simulink model "q2x2sim"  (R2025b)
settings: Solver=ode45  StartTime=0.0  StopTime=15  MaxStep=.1  RelTol=1e-6  AbsTol=1e-6
model workspace (MAT data in the model file):
  Omega = 0.6
values from neighbouring files (symbols this model uses):
  A = zeros(sum(neqs), 4*NK)    [kernelsc.m]    (also in kernelscinv.m; kernelso.m; kernelsoinv.m; q2x2simu.m = zeros(2*xg))
  Ao = A - [P1; P2]*C    [q2x2simu.m]
  B = zeros(2*xg, 1)    [q2x2simu.m]
  Bo = [[P1; P2] + r*B, B]    [q2x2simu.m]
  C = B'    [q2x2simu.m]
  mu0 = 8    [bounds.m]    (also in histogrametc.m = 10; q2x2simu.m)
  xg = 128    [bounds.m]    (also in q2x2simu.m)
  z0 = [p * v0_ic(x1); v0_ic(x0)]    [histogrametc.m]    (also in q2x2simu.m = [p*v0(x1), v0(x0)]')
  z0hat = 1.5 * z0    [histogrametc.m]    (also in q2x2simu.m = 1.5*z0)
undefined symbols (not defined in the file or in its folder): K1, K2
settings Model: Creator=humaloja  LastModifiedBy=koudohodeflorent

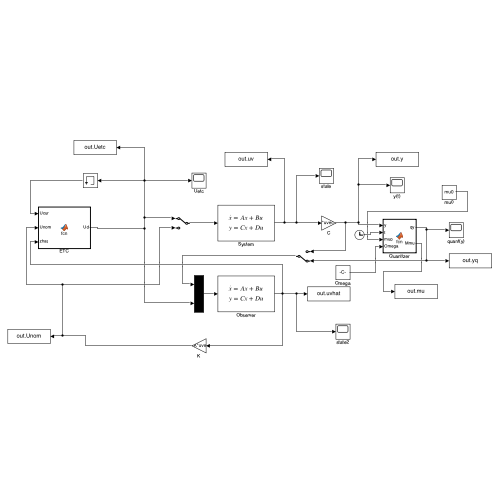
[thumbnail: Simulink's stored preview of the top-level diagram]
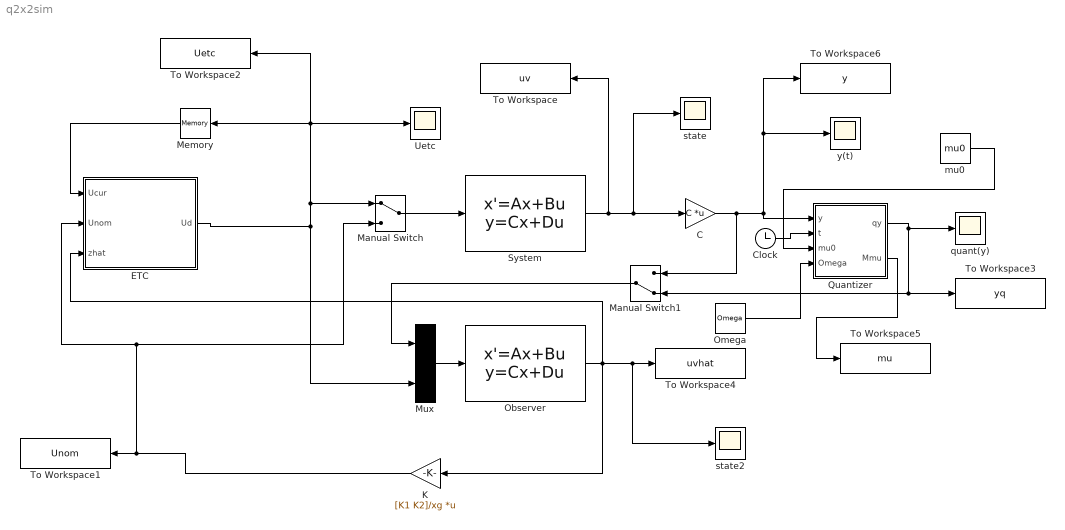
== system q2x2sim ==
  C : Gain  Gain=C  Multiplication=Matrix(K*u) (u vector)
  Clock : Clock
  ETC : MATLAB Function  TreatAsAtomicUnit=on
  K : Gain  Gain=[K1 K2]/xg  Multiplication=Matrix(K*u) (u vector)
  Manual Switch : ManualSwitch
  Manual Switch1 : ManualSwitch  CurrentSetting=0
  Memory : Memory
  Mux : Mux  Inputs=2
  Observer : StateSpace  A=Ao  B=Bo  C=eye(2*xg)  D=zeros(2*xg,2)  InitialCondition=z0hat
  Omega : Constant  Value=Omega
  Quantizer : MATLAB Function  TreatAsAtomicUnit=on
  System : StateSpace  A=A  B=B  C=eye(2*xg)  D=zeros(2*xg,1)  InitialCondition=z0
  To Workspace : ToWorkspace  VariableName=uv  SaveFormat=Timeseries  SampleTime=-1
  To Workspace1 : ToWorkspace  VariableName=Unom  SaveFormat=Timeseries  SampleTime=-1
  To Workspace2 : ToWorkspace  VariableName=Uetc  SaveFormat=Timeseries  SampleTime=-1
  To Workspace3 : ToWorkspace  VariableName=yq  SaveFormat=Timeseries  SampleTime=-1
  To Workspace4 : ToWorkspace  VariableName=uvhat  SaveFormat=Timeseries  SampleTime=-1
  To Workspace5 : ToWorkspace  VariableName=mu  SaveFormat=Timeseries  SampleTime=-1
  To Workspace6 : ToWorkspace  VariableName=y  SaveFormat=Timeseries  SampleTime=-1
  Uetc : Scope
      settings: ActiveDisplayYMinimum=-1  ActiveDisplayYMaximum=1
  mu0 : Constant  Value=mu0
  quant(y) : Scope
      settings: ActiveDisplayYMinimum=-10.5  ActiveDisplayYMaximum=4.5  DataLoggingVariableName=ScopeData2
  state : Scope
      settings: ActiveDisplayYMinimum=-1  ActiveDisplayYMaximum=1  DataLoggingVariableName=ScopeData4
  state2 : Scope
      settings: ActiveDisplayYMinimum=-20.70698  ActiveDisplayYMaximum=18.96744
  y(t) : Scope
      settings: ActiveDisplayYMinimum=-1  ActiveDisplayYMaximum=1
  wires:
  Mux/1 -> Observer/1
  System/1 -> To Workspace/1, state/1, C/1
  Quantizer/1(qy) -> quant(y)/1, Manual Switch1/2, To Workspace3/1
  Clock/1 -> Quantizer/2(t)
  Observer/1 -> K/1, ETC/3(zhat), state2/1, To Workspace4/1
  ETC/1(Ud) -> To Workspace2/1, Uetc/1, Memory/1, Manual Switch/1, Mux/2
  Quantizer/2(Mmu) -> To Workspace5/1
  K/1 -> Manual Switch/2, ETC/2(Unom), To Workspace1/1
  Memory/1 -> ETC/1(Ucur)
  Manual Switch/1 -> System/1
  C/1 -> Manual Switch1/1, To Workspace6/1, y(t)/1, Quantizer/1(y)
  Manual Switch1/1 -> Mux/1
  mu0/1 -> Quantizer/3(mu0)
  Omega/1 -> Quantizer/4(Omega)

== matlab function q2x2sim/Quantizer ==
  data: y input; qy output; t input; Mmu output; mu0 input; Omega input
function [qy, Mmu] = fcn(y,t,mu0,Omega)
% parameters
M = 3; Delta = M/10 ; T = 2;
   % mu0 =1; Omega =1; T = 2;
   % mu0 =15; Omega =1; T = 2;

% mu
mu = mu0*Omega^floor(t/T);
Mmu = M*mu;

% quantizer
if y/mu > M
  qy = M;
elseif y/mu < -M
  qy = -M;
else
  qy = Delta*floor(y/(mu*Delta) + 0.5);
end
% multiply output by mu
qy = mu*qy;

% FOR TESTING: disable quantization by just returning y
%qy = y;
end

== matlab function q2x2sim/ETC ==
  data: Ucur input; Unom input; Ud output; zhat input
function Ud  = fcn(Ucur, Unom, zhat)
% parameters
Cetm = 0.14;
wk   = 0;

% split zhat to uhat and vhat
xg = numel(zhat)/2;

if abs(Unom - Ucur) > Cetm*(norm(zhat(1:xg),inf) + norm(zhat(xg+1:2*xg),inf) + wk)
    Ud        = Unom;
else
    Ud        = Ucur;
    wk        = norm(zhat(1:xg),inf) + norm(zhat(xg+1:2*xg),inf);
end
end
